simulink model "servomotor_p_feedforward"  (R2020b)
settings: Solver=VariableStepAuto  StartTime=0.0  StopTime=tempoSimulacao  RelTol=1e-3
values from neighbouring files (symbols this model uses):
  controlador = projetarControladorPI(planta, requisitos)    [avaliarIndutor.m]
  planta = obterPlantaServo()    [avaliarIndutor.m]
undefined symbols (not defined in the file or in its folder): disturbio, referencia
settings Model: Creator=mmaximo  LastModifiedBy=rudog

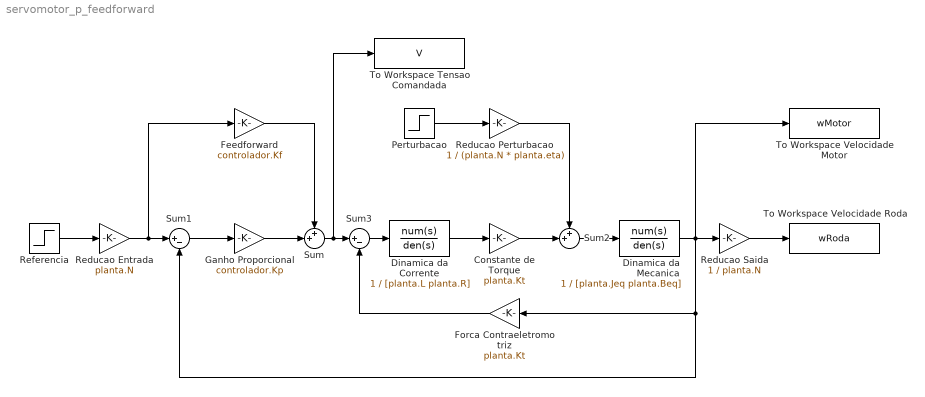
== system servomotor_p_feedforward ==
  Constante de Torque : Gain  Gain=planta.Kt
  Dinamica da Corrente : TransferFcn  Numerator=1  Denominator=[planta.L planta.R]
  Dinamica da Mecanica : TransferFcn  Numerator=1  Denominator=[planta.Jeq planta.Beq]
  Feedforward : Gain  Gain=controlador.Kf
  Forca Contraeletromotriz : Gain  Gain=planta.Kt
  Ganho Proporcional : Gain  Gain=controlador.Kp
  Perturbacao : Step  Time=disturbio.instante  After=disturbio.amplitude  SampleTime=0
  Reducao Entrada : Gain  Gain=planta.N
  Reducao Perturbacao : Gain  Gain=1 / (planta.N * planta.eta)
  Reducao Saida : Gain  Gain=1 / planta.N
  Referencia : Step  Time=referencia.instante  After=referencia.amplitude  SampleTime=0
  Sum : Sum  Inputs=++|
  Sum1 : Sum  Inputs=|+-
  Sum2 : Sum  Inputs=++|
  Sum3 : Sum  Inputs=|+-
  To Workspace Tensao Comandada : ToWorkspace  VariableName=V  SaveFormat=Structure With Time  SampleTime=-1
  To Workspace Velocidade Motor : ToWorkspace  VariableName=wMotor  SaveFormat=Structure With Time  SampleTime=-1
  To Workspace Velocidade Roda : ToWorkspace  VariableName=wRoda  SaveFormat=Structure With Time  SampleTime=-1
  wires:
  Perturbacao/1 -> Reducao Perturbacao/1
  Dinamica da Corrente/1 -> Constante de Torque/1
  Dinamica da Mecanica/1 -> Reducao Saida/1, Sum1/2, Forca Contraeletromotriz/1, To Workspace Velocidade Motor/1
  Referencia/1 -> Reducao Entrada/1
  Reducao Saida/1 -> To Workspace Velocidade Roda/1
  Reducao Entrada/1 -> Feedforward/1, Sum1/1
  Reducao Perturbacao/1 -> Sum2/1
  Sum1/1 -> Ganho Proporcional/1
  Constante de Torque/1 -> Sum2/2
  Sum2/1 -> Dinamica da Mecanica/1
  Ganho Proporcional/1 -> Sum/2
  Feedforward/1 -> Sum/1
  Sum/1 -> To Workspace Tensao Comandada/1, Sum3/1
  Sum3/1 -> Dinamica da Corrente/1
  Forca Contraeletromotriz/1 -> Sum3/2
